simulink model "CLFeedbackObserver"  (R2021b)
settings: Solver=VariableStepAuto  StartTime=0.0  StopTime=10.0  RelTol=1e-3
values from neighbouring files (symbols this model uses):
  D = double(D)    [Main.m]
  F = inv(CMin*inv(-AMin+BMin*K)*BMin)    [Main.m]
  N1 = double(N1)    [Main.m]
  N2 = double(N2)    [Main.m]
undefined symbols (not defined in the file or in its folder): AMin, BMin, CMin, DMin, tau_threshold
settings Model: Creator=angelhoffman  LastModifiedBy=William Watkins
settings DebuggingCC: UnconnectedInputMsg=none  UnconnectedOutputMsg=none  UnconnectedLineMsg=none
settings RTWCC: DLArmComputeVersion=20.02.1

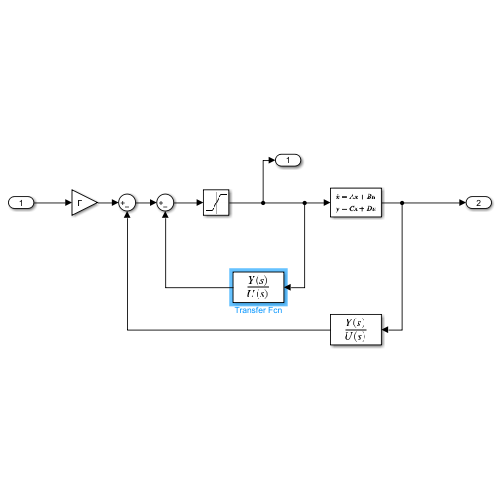
[thumbnail: Simulink's stored preview of the top-level diagram]
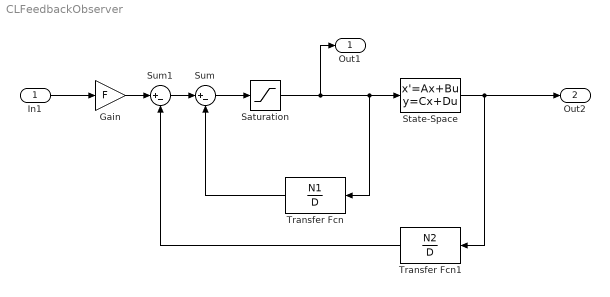
== system CLFeedbackObserver ==
  In1 : Inport
  Gain : Gain  Gain=F
  Saturation : Saturate  UpperLimit=tau_threshold  LowerLimit=-tau_threshold
  State-Space : StateSpace  A=AMin  B=BMin  C=CMin  D=DMin  InitialCondition=zeros(4,1)
  Sum : Sum  Inputs=|+-
  Sum1 : Sum  Inputs=|+-
  Transfer Fcn : TransferFcn  Numerator=N1  Denominator=D
  Transfer Fcn1 : TransferFcn  Numerator=N2  Denominator=D
  Out1 : Outport
  Out2 : Outport  Port=2
  wires:
  State-Space/1 -> Out2/1, Transfer Fcn1/1
  Sum/1 -> Saturation/1
  Saturation/1 -> Out1/1, Transfer Fcn/1, State-Space/1
  In1/1 -> Gain/1
  Transfer Fcn/1 -> Sum/2
  Transfer Fcn1/1 -> Sum1/2
  Gain/1 -> Sum1/1
  Sum1/1 -> Sum/1
